simulink model "CRH2forBenchmark_Copy"  (R2014a)
settings: Solver=ode3  StartTime=0.0  StopTime=1  FixedStep=1e-5  RelTol=1e-3
PostLoadFcn:
  | , if any(exist('dsrtsu_mdlpostloadfcn', 'file') == [2, 3, 6]), try dsrtsu_mdlpostloadfcn('Execute', bdroot); catch fprintf('Error in PostLoadFcn (dsrtsu_mdlpostloadfcn) for model "%s":\n %s\n', bdroot, lasterr); end, end,
values from neighbouring files (symbols this model uses):
  Cd = 0.016    [CRH2forBenchmark.mat]
  Lm = 0.032848    [CRH2forBenchmark.mat]
  Ln = 0.002    [CRH2forBenchmark.mat]
  Lr = 0.034142    [CRH2forBenchmark.mat]
  Ls = 0.0342654    [CRH2forBenchmark.mat]
  np = 2    [CRH2forBenchmark.mat]
  Rd = 6000    [CRH2forBenchmark.mat]
  Rn = 0.2    [CRH2forBenchmark.mat]
  Rr = 0.146    [CRH2forBenchmark.mat]
  Rs = 0.144    [CRH2forBenchmark.mat]
  ts = 1e-05    [CRH2forBenchmark.mat]
undefined symbols (not defined in the file): J, KIM, KIT, KPM, KPT, phir, Ts, Vge
libraries: simulink x20
(part 3 of 5)

== system CRH2forBenchmark_Copy/Benchmark/SFI2/Subsystem ==
  Normal : Inport
  Outside Signal : Inport  Port=2
  Band-Limited White Noise : simulink/Sources/Band-Limited White Noise  Cov=NoiseFault(1)  Ts=NoiseFault(2)  seed=NoiseFault(3)
  Pulse Generator : DiscretePulseGenerator  PulseType=Time based  Amplitude=PeriodicFault(1)  Period=PeriodicFault(2)  PulseWidth=PeriodicFault(3)
  SFI1 : Subsystem  mask{sfcnParam1=AddMux, sfcnParam2=Comp_ConV, sfcnParam3=DriftFault, sfcnParam4=FaultCont, sfcnParam5=FaultInjectionTime, sfcnParam6=FaultType, sfcnParam7=NoiseSelec, sfcnParam8=ShockGain, sfcnParam9=Variance}
      mask prompts: sfcnParam1 "AddMux:"; sfcnParam2 "Comp_ConV:"; sfcnParam3 "DriftFault:"; sfcnParam4 "FaultCont:"; sfcnParam5 "FaultInjectionTime:"; sfcnParam6 "FaultType:"; sfcnParam7 "NoiseSelec:"; sfcnParam8 "ShockGain:"; sfcnParam9 "Variance:"
      mask help: Simulink:masks:GenSFuncDesc_MD
      mask Help: eval('feval(''rtwprivate'',''rtwhelpview'',''rtw_sfcn_block'')');
  Out : Outport
  tag scope: BandLimitedWhiteNoiseSFI2=global, PulseGeneratorSFI2=global
  wires:
  Band-Limited White Noise/1 -> [BandLimitedWhiteNoiseSFI2]
  Pulse Generator/1 -> [PulseGeneratorSFI2]
  Normal/1 -> SFI1/1(Nomal)
  Outside Signal/1 -> SFI1/2(Outside Signal)
  SFI1/1(Out) -> Out/1

== system CRH2forBenchmark_Copy/Benchmark/TFI1/TFI1Sub ==
  Nomal : Inport
  Outside Signal : Inport  Port=2
  Add : Sum
  Band-Limited White Noise : simulink/Sources/Band-Limited White Noise  Cov=NoiseFault(1)  Ts=NoiseFault(2)  seed=NoiseFault(3)
  Logic Operation : Subsystem
  Noise0 : Constant  Value=0
  NoiseAdd : Sum  Inputs=++|
  NoiseSelec : Constant  Value=NoiseSelec
  Product : Product
  Switch : Switch  Criteria=u2 ~= 0
  TFI : Subsystem
  Out : Outport
  wires:
  Outside Signal/1 -> TFI/1(Outside Signal)
  Switch/1 -> NoiseAdd/1
  Band-Limited White Noise/1 -> Switch/1
  [Fault] -> Logic Operation/5(Fault), Add/2, Product/2
  NoiseAdd/1 -> Out/1
  Logic Operation/1(Out) -> NoiseAdd/2
  Nomal/1 -> Add/1, Product/1, Logic Operation/4(Normal)
  Add/1 -> Logic Operation/2(Add)
  Noise0/1 -> Switch/3
  TFI/1(Fault Singal) -> [Fault]
  Product/1 -> Logic Operation/3(Mux)
  TFI/2(Selector) -> [Selector]
  [Selector] -> Logic Operation/1(Selector)
  NoiseSelec/1 -> Switch/2

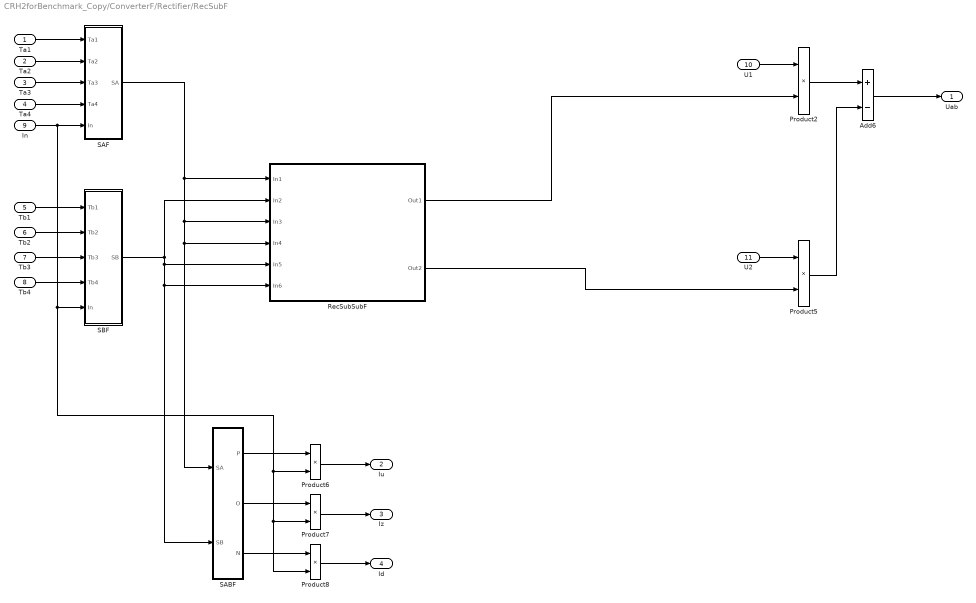
== system CRH2forBenchmark_Copy/ConverterF/Rectifier/RecSubF ==
  Ta1 : Inport
  Ta2 : Inport  Port=2
  Ta3 : Inport  Port=3
  Ta4 : Inport  Port=4
  Tb1 : Inport  Port=5
  Tb2 : Inport  Port=6
  Tb3 : Inport  Port=7
  Tb4 : Inport  Port=8
  In : Inport  Port=9
  U1 : Inport  Port=10
  U2 : Inport  Port=11
  Add6 : Sum  Inputs=+-  SampleTime=ts
  Product{2,5..8} (5 alike) : Product  SampleTime=ts
  RecSubSubF : Subsystem
      mask help: Simulink:masks:GenSFuncDesc_MD
      mask Help: eval('feval(''rtwprivate'',''rtwhelpview'',''rtw_sfcn_block'')');
  SABF : Subsystem
      mask help: Simulink:masks:GenSFuncDesc_MD
      mask Help: eval('feval(''rtwprivate'',''rtwhelpview'',''rtw_sfcn_block'')');
  SAF : Subsystem
      mask help: Simulink:masks:GenSFuncDesc_MD
      mask Help: eval('feval(''rtwprivate'',''rtwhelpview'',''rtw_sfcn_block'')');
  SBF : Subsystem
      mask help: Simulink:masks:GenSFuncDesc_MD
      mask Help: eval('feval(''rtwprivate'',''rtwhelpview'',''rtw_sfcn_block'')');
  Uab : Outport
  Iu : Outport  Port=2
  Iz : Outport  Port=3
  Id : Outport  Port=4
  wires:
  In/1 -> SAF/5(In), SBF/5(In), Product7/2, Product8/2, Product6/2
  Tb3/1 -> SBF/3(Tb3)
  U2/1 -> Product5/1
  Product2/1 -> Add6/1
  SAF/1(SA) -> RecSubSubF/1(In1), RecSubSubF/3(In3), RecSubSubF/4(In4), SABF/1(SA)
  U1/1 -> Product2/1
  Ta3/1 -> SAF/3(Ta3)
  Product5/1 -> Add6/2
  Tb1/1 -> SBF/1(Tb1)
  Add6/1 -> Uab/1
  Ta2/1 -> SAF/2(Ta2)
  Tb2/1 -> SBF/2(Tb2)
  SBF/1(SB) -> RecSubSubF/2(In2), RecSubSubF/5(In5), RecSubSubF/6(In6), SABF/2(SB)
  Tb4/1 -> SBF/4(Tb4)
  Ta1/1 -> SAF/1(Ta1)
  Ta4/1 -> SAF/4(Ta4)
  SABF/3(N) -> Product8/1
  SABF/2(O) -> Product7/1
  SABF/1(P) -> Product6/1
  Product6/1 -> Iu/1
  Product7/1 -> Iz/1
  Product8/1 -> Id/1
  RecSubSubF/1(Out1) -> Product2/2
  RecSubSubF/2(Out2) -> Product5/2

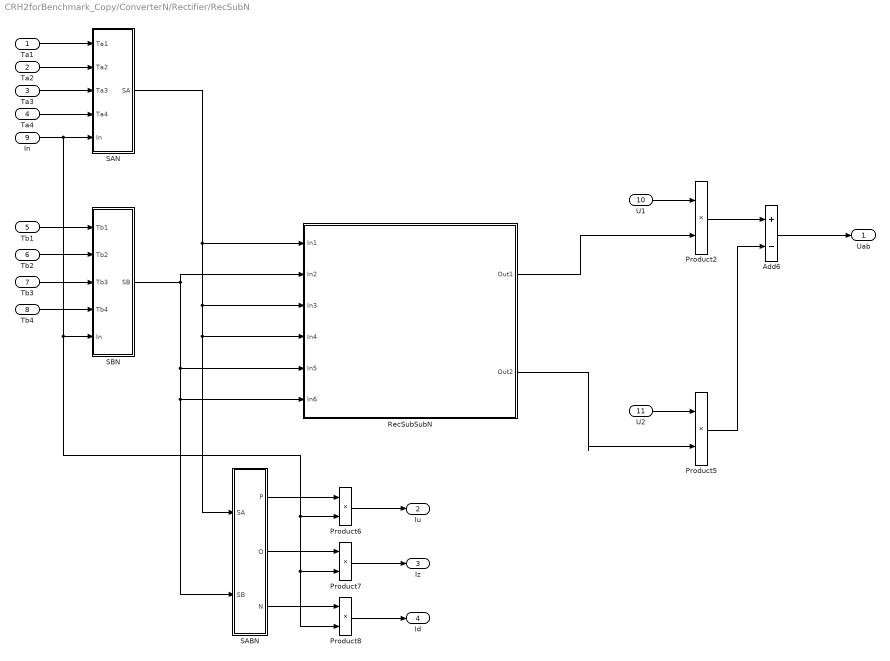
== system CRH2forBenchmark_Copy/ConverterN/Rectifier/RecSubN ==
  Ta1 : Inport
  Ta2 : Inport  Port=2
  Ta3 : Inport  Port=3
  Ta4 : Inport  Port=4
  Tb1 : Inport  Port=5
  Tb2 : Inport  Port=6
  Tb3 : Inport  Port=7
  Tb4 : Inport  Port=8
  In : Inport  Port=9
  U1 : Inport  Port=10
  U2 : Inport  Port=11
  Add6 : Sum  Inputs=+-  SampleTime=ts
  Product{2,5..8} (5 alike) : Product  SampleTime=ts
  RecSubSubN : Subsystem
      mask help: Simulink:masks:GenSFuncDesc_MD
      mask Help: eval('feval(''rtwprivate'',''rtwhelpview'',''rtw_sfcn_block'')');
  SABN : Subsystem
      mask help: Simulink:masks:GenSFuncDesc_MD
      mask Help: eval('feval(''rtwprivate'',''rtwhelpview'',''rtw_sfcn_block'')');
  SAN : Subsystem
      mask help: Simulink:masks:GenSFuncDesc_MD
      mask Help: eval('feval(''rtwprivate'',''rtwhelpview'',''rtw_sfcn_block'')');
  SBN : Subsystem
      mask help: Simulink:masks:GenSFuncDesc_MD
      mask Help: eval('feval(''rtwprivate'',''rtwhelpview'',''rtw_sfcn_block'')');
  Uab : Outport
  Iu : Outport  Port=2
  Iz : Outport  Port=3
  Id : Outport  Port=4
  wires:
  Product8/1 -> Id/1
  Product7/1 -> Iz/1
  Product6/1 -> Iu/1
  SABN/1(P) -> Product6/1
  SABN/2(O) -> Product7/1
  SABN/3(N) -> Product8/1
  Ta4/1 -> SAN/4(Ta4)
  Ta1/1 -> SAN/1(Ta1)
  Tb4/1 -> SBN/4(Tb4)
  SBN/1(SB) -> RecSubSubN/2(In2), RecSubSubN/5(In5), RecSubSubN/6(In6), SABN/2(SB)
  Tb2/1 -> SBN/2(Tb2)
  Ta2/1 -> SAN/2(Ta2)
  Add6/1 -> Uab/1
  Tb1/1 -> SBN/1(Tb1)
  Product5/1 -> Add6/2
  Ta3/1 -> SAN/3(Ta3)
  U1/1 -> Product2/1
  SAN/1(SA) -> RecSubSubN/1(In1), RecSubSubN/3(In3), RecSubSubN/4(In4), SABN/1(SA)
  Product2/1 -> Add6/1
  U2/1 -> Product5/1
  Tb3/1 -> SBN/3(Tb3)
  In/1 -> SAN/5(In), SBN/5(In), Product6/2, Product8/2, Product7/2
  RecSubSubN/1(Out1) -> Product2/2
  RecSubSubN/2(Out2) -> Product5/2

== system CRH2forBenchmark_Copy/InverterF/InverterTuF/__InputSSForSFun__ ==
  Tu1 : Inport
  Tu2 : Inport  Port=2
  Tu3 : Inport  Port=3
  Tu4 : Inport  Port=4
  Ia : Inport  Port=5
  U1 : Inport  Port=6
  U2 : Inport  Port=7
  __UniqueOutportName__1__ : Outport
  __UniqueOutportName__2__ : Outport  Port=2
  __UniqueOutportName__3__ : Outport  Port=3
  __UniqueOutportName__4__ : Outport  Port=4
  __UniqueOutportName__5__ : Outport  Port=5
  __UniqueOutportName__6__ : Outport  Port=6
  __UniqueOutportName__7__ : Outport  Port=7
  wires:
  Tu1/1 -> __UniqueOutportName__1__/1
  Tu2/1 -> __UniqueOutportName__2__/1
  Tu3/1 -> __UniqueOutportName__3__/1
  Tu4/1 -> __UniqueOutportName__4__/1
  Ia/1 -> __UniqueOutportName__5__/1
  U1/1 -> __UniqueOutportName__6__/1
  U2/1 -> __UniqueOutportName__7__/1

== system CRH2forBenchmark_Copy/InverterF/InverterTuF/__OutputSSForSFun__ ==
  __UniqueInportName__1__ : Inport
  __UniqueInportName__2__ : Inport  Port=2
  __UniqueInportName__3__ : Inport  Port=3
  __UniqueInportName__4__ : Inport  Port=4
  Iu : Outport
  Iz : Outport  Port=2
  Id : Outport  Port=3
  Vu : Outport  Port=4
  wires:
  __UniqueInportName__1__/1 -> Iu/1
  __UniqueInportName__2__/1 -> Iz/1
  __UniqueInportName__3__/1 -> Id/1
  __UniqueInportName__4__/1 -> Vu/1

== system CRH2forBenchmark_Copy/InverterF/InverterTvF/__InputSSForSFun__ ==
  Tv1 : Inport
  Tv2 : Inport  Port=2
  Tv3 : Inport  Port=3
  Tv4 : Inport  Port=4
  Ib : Inport  Port=5
  U1 : Inport  Port=6
  U2 : Inport  Port=7
  __UniqueOutportName__1__ : Outport
  __UniqueOutportName__2__ : Outport  Port=2
  __UniqueOutportName__3__ : Outport  Port=3
  __UniqueOutportName__4__ : Outport  Port=4
  __UniqueOutportName__5__ : Outport  Port=5
  __UniqueOutportName__6__ : Outport  Port=6
  __UniqueOutportName__7__ : Outport  Port=7
  wires:
  Tv1/1 -> __UniqueOutportName__1__/1
  Tv2/1 -> __UniqueOutportName__2__/1
  Tv3/1 -> __UniqueOutportName__3__/1
  Tv4/1 -> __UniqueOutportName__4__/1
  Ib/1 -> __UniqueOutportName__5__/1
  U1/1 -> __UniqueOutportName__6__/1
  U2/1 -> __UniqueOutportName__7__/1

== system CRH2forBenchmark_Copy/InverterF/InverterTvF/__OutputSSForSFun__ ==
  __UniqueInportName__1__ : Inport
  __UniqueInportName__2__ : Inport  Port=2
  __UniqueInportName__3__ : Inport  Port=3
  __UniqueInportName__4__ : Inport  Port=4
  Iu : Outport
  Iz : Outport  Port=2
  Id : Outport  Port=3
  Vv : Outport  Port=4
  wires:
  __UniqueInportName__1__/1 -> Iu/1
  __UniqueInportName__2__/1 -> Iz/1
  __UniqueInportName__3__/1 -> Id/1
  __UniqueInportName__4__/1 -> Vv/1

== system CRH2forBenchmark_Copy/InverterF/InverterTwF/__InputSSForSFun__ ==
  Tw1 : Inport
  Tw2 : Inport  Port=2
  Tw3 : Inport  Port=3
  Tw4 : Inport  Port=4
  Ic : Inport  Port=5
  U1 : Inport  Port=6
  U2 : Inport  Port=7
  __UniqueOutportName__1__ : Outport
  __UniqueOutportName__2__ : Outport  Port=2
  __UniqueOutportName__3__ : Outport  Port=3
  __UniqueOutportName__4__ : Outport  Port=4
  __UniqueOutportName__5__ : Outport  Port=5
  __UniqueOutportName__6__ : Outport  Port=6
  __UniqueOutportName__7__ : Outport  Port=7
  wires:
  Tw1/1 -> __UniqueOutportName__1__/1
  Tw2/1 -> __UniqueOutportName__2__/1
  Tw3/1 -> __UniqueOutportName__3__/1
  Tw4/1 -> __UniqueOutportName__4__/1
  Ic/1 -> __UniqueOutportName__5__/1
  U1/1 -> __UniqueOutportName__6__/1
  U2/1 -> __UniqueOutportName__7__/1

== system CRH2forBenchmark_Copy/InverterF/InverterTwF/__OutputSSForSFun__ ==
  __UniqueInportName__1__ : Inport
  __UniqueInportName__2__ : Inport  Port=2
  __UniqueInportName__3__ : Inport  Port=3
  __UniqueInportName__4__ : Inport  Port=4
  Iu : Outport
  Iz : Outport  Port=2
  Id : Outport  Port=3
  Vw : Outport  Port=4
  wires:
  __UniqueInportName__1__/1 -> Iu/1
  __UniqueInportName__2__/1 -> Iz/1
  __UniqueInportName__3__/1 -> Id/1
  __UniqueInportName__4__/1 -> Vw/1

== system CRH2forBenchmark_Copy/InverterN/InverterTuN/__InputSSForSFun__ ==
  Tu1 : Inport
  Tu2 : Inport  Port=2
  Tu3 : Inport  Port=3
  Tu4 : Inport  Port=4
  Ia : Inport  Port=5
  U1 : Inport  Port=6
  U2 : Inport  Port=7
  __UniqueOutportName__1__ : Outport
  __UniqueOutportName__2__ : Outport  Port=2
  __UniqueOutportName__3__ : Outport  Port=3
  __UniqueOutportName__4__ : Outport  Port=4
  __UniqueOutportName__5__ : Outport  Port=5
  __UniqueOutportName__6__ : Outport  Port=6
  __UniqueOutportName__7__ : Outport  Port=7
  wires:
  Tu1/1 -> __UniqueOutportName__1__/1
  Tu2/1 -> __UniqueOutportName__2__/1
  Tu3/1 -> __UniqueOutportName__3__/1
  Tu4/1 -> __UniqueOutportName__4__/1
  Ia/1 -> __UniqueOutportName__5__/1
  U1/1 -> __UniqueOutportName__6__/1
  U2/1 -> __UniqueOutportName__7__/1

== system CRH2forBenchmark_Copy/InverterN/InverterTuN/__OutputSSForSFun__ ==
  __UniqueInportName__1__ : Inport
  __UniqueInportName__2__ : Inport  Port=2
  __UniqueInportName__3__ : Inport  Port=3
  __UniqueInportName__4__ : Inport  Port=4
  Iu : Outport
  Iz : Outport  Port=2
  Id : Outport  Port=3
  Vu : Outport  Port=4
  wires:
  __UniqueInportName__1__/1 -> Iu/1
  __UniqueInportName__2__/1 -> Iz/1
  __UniqueInportName__3__/1 -> Id/1
  __UniqueInportName__4__/1 -> Vu/1

== system CRH2forBenchmark_Copy/InverterN/InverterTvN/__InputSSForSFun__ ==
  Tv1 : Inport
  Tv2 : Inport  Port=2
  Tv3 : Inport  Port=3
  Tv4 : Inport  Port=4
  Ib : Inport  Port=5
  U1 : Inport  Port=6
  U2 : Inport  Port=7
  __UniqueOutportName__1__ : Outport
  __UniqueOutportName__2__ : Outport  Port=2
  __UniqueOutportName__3__ : Outport  Port=3
  __UniqueOutportName__4__ : Outport  Port=4
  __UniqueOutportName__5__ : Outport  Port=5
  __UniqueOutportName__6__ : Outport  Port=6
  __UniqueOutportName__7__ : Outport  Port=7
  wires:
  Tv1/1 -> __UniqueOutportName__1__/1
  Tv2/1 -> __UniqueOutportName__2__/1
  Tv3/1 -> __UniqueOutportName__3__/1
  Tv4/1 -> __UniqueOutportName__4__/1
  Ib/1 -> __UniqueOutportName__5__/1
  U1/1 -> __UniqueOutportName__6__/1
  U2/1 -> __UniqueOutportName__7__/1

== system CRH2forBenchmark_Copy/InverterN/InverterTvN/__OutputSSForSFun__ ==
  __UniqueInportName__1__ : Inport
  __UniqueInportName__2__ : Inport  Port=2
  __UniqueInportName__3__ : Inport  Port=3
  __UniqueInportName__4__ : Inport  Port=4
  Iu : Outport
  Iz : Outport  Port=2
  Id : Outport  Port=3
  Vv : Outport  Port=4
  wires:
  __UniqueInportName__1__/1 -> Iu/1
  __UniqueInportName__2__/1 -> Iz/1
  __UniqueInportName__3__/1 -> Id/1
  __UniqueInportName__4__/1 -> Vv/1

== system CRH2forBenchmark_Copy/InverterN/InverterTwN/__InputSSForSFun__ ==
  Tw1 : Inport
  Tw2 : Inport  Port=2
  Tw3 : Inport  Port=3
  Tw4 : Inport  Port=4
  Ic : Inport  Port=5
  U1 : Inport  Port=6
  U2 : Inport  Port=7
  __UniqueOutportName__1__ : Outport
  __UniqueOutportName__2__ : Outport  Port=2
  __UniqueOutportName__3__ : Outport  Port=3
  __UniqueOutportName__4__ : Outport  Port=4
  __UniqueOutportName__5__ : Outport  Port=5
  __UniqueOutportName__6__ : Outport  Port=6
  __UniqueOutportName__7__ : Outport  Port=7
  wires:
  Tw1/1 -> __UniqueOutportName__1__/1
  Tw2/1 -> __UniqueOutportName__2__/1
  Tw3/1 -> __UniqueOutportName__3__/1
  Tw4/1 -> __UniqueOutportName__4__/1
  Ic/1 -> __UniqueOutportName__5__/1
  U1/1 -> __UniqueOutportName__6__/1
  U2/1 -> __UniqueOutportName__7__/1

== system CRH2forBenchmark_Copy/InverterN/InverterTwN/__OutputSSForSFun__ ==
  __UniqueInportName__1__ : Inport
  __UniqueInportName__2__ : Inport  Port=2
  __UniqueInportName__3__ : Inport  Port=3
  __UniqueInportName__4__ : Inport  Port=4
  Iu : Outport
  Iz : Outport  Port=2
  Id : Outport  Port=3
  Vw : Outport  Port=4
  wires:
  __UniqueInportName__1__/1 -> Iu/1
  __UniqueInportName__2__/1 -> Iz/1
  __UniqueInportName__3__/1 -> Id/1
  __UniqueInportName__4__/1 -> Vw/1

== system CRH2forBenchmark_Copy/Machine model/Normal ModelF/MeasurementF ==
  isα : Inport
  isβ : Inport  Port=2
  irα : Inport  Port=3
  irβ : Inport  Port=4
  TL : Inport  Port=5
  MeasurementF_sfcn : S-Function  FunctionName=MeasurementF_sf  Parameters=sfcnParam1, sfcnParam2, sfcnParam3  SFunctionModules=""  EnableBusSupport=off  mask{rtw_sf_name=MeasurementF_sf, showVar=off, sfcnParam1=sfcnParam1, sfcnParam2=sfcnParam2, sfcnParam3=sfcnParam3}
      mask prompts: rtw_sf_name "Simulink:masks:GenSFuncName_MP"; showVar "Simulink:masks:GenSFuncShowModuleList_MP"; sfcnParam1 "J:"; sfcnParam2 "Lm:"; sfcnParam3 "np:"
      mask help: Simulink:masks:GenSFuncDesc_MD
      mask init: same as CRH2forBenchmark_Copy/DCU1/DCU1_sfcn
      settings: CopyFcn=|
      | if ~strcmp(get_param(gcb,'Linkstatus'),'none') && ...
      | ~strcmp(get_param(gcb,'Linkstatus'),'implicit')
      |   set_param(gcb,'LinkStatus','none');
      | end
      mask Help: eval('feval(''rtwprivate'',''rtwhelpview'',''rtw_sfcn_block'')');
      mask Display:
      | port_label('input',1,'isα');
      | port_label('input',2,'isβ');
      | port_label('input',3,'irα');
      | port_label('input',4,'irβ');
      | port_label('input',5,'TL');
      | port_label('output',1,'Te');
      | port_label('output',2,'ω');
      | port_label('output',3,'Isabc');
  __InputSSForSFun__ : Subsystem
  __OutputSSForSFun__ : Subsystem
  Te : Outport
  ω : Outport  Port=2
  Isabc : Outport  Port=3
  wires:
  isα/1 -> __InputSSForSFun__/1(isα)
  isβ/1 -> __InputSSForSFun__/2(isβ)
  irα/1 -> __InputSSForSFun__/3(irα)
  irβ/1 -> __InputSSForSFun__/4(irβ)
  TL/1 -> __InputSSForSFun__/5(TL)
  __InputSSForSFun__/1(__UniqueOutportName__1__) -> MeasurementF_sfcn/1
  __InputSSForSFun__/2(__UniqueOutportName__2__) -> MeasurementF_sfcn/2
  __InputSSForSFun__/3(__UniqueOutportName__3__) -> MeasurementF_sfcn/3
  __InputSSForSFun__/4(__UniqueOutportName__4__) -> MeasurementF_sfcn/4
  __InputSSForSFun__/5(__UniqueOutportName__5__) -> MeasurementF_sfcn/5
  MeasurementF_sfcn/1 -> __OutputSSForSFun__/1(__UniqueInportName__1__)
  MeasurementF_sfcn/2 -> __OutputSSForSFun__/2(__UniqueInportName__2__)
  MeasurementF_sfcn/3 -> __OutputSSForSFun__/3(__UniqueInportName__3__)
  __OutputSSForSFun__/1(Te) -> Te/1
  __OutputSSForSFun__/2(ω) -> ω/1
  __OutputSSForSFun__/3(Isabc) -> Isabc/1

== system CRH2forBenchmark_Copy/Machine model/Normal ModelF/MotorSubsystem1F ==
  ψrβ : Inport
  Usβ : Inport  Port=2
  MotorSubsystem1FSub : Subsystem
  isβ : Outport
  ψsβ : Outport  Port=2
  wires:
  ψrβ/1 -> MotorSubsystem1FSub/1(ψrβ)
  Usβ/1 -> MotorSubsystem1FSub/2(Usβ)
  MotorSubsystem1FSub/1(isβ) -> isβ/1
  MotorSubsystem1FSub/2(ψsβ) -> ψsβ/1

== system CRH2forBenchmark_Copy/Machine model/Normal ModelF/MotorSubsystem2F ==
  ψsα : Inport
  ψrβ : Inport  Port=2
  ω : Inport  Port=3
  MotorSubsystem2FSub : Subsystem
  irα : Outport
  ψrα : Outport  Port=2
  wires:
  ψsα/1 -> MotorSubsystem2FSub/1(ψsα)
  ψrβ/1 -> MotorSubsystem2FSub/2(ψrβ)
  ω/1 -> MotorSubsystem2FSub/3(ω)
  MotorSubsystem2FSub/1(irα) -> irα/1
  MotorSubsystem2FSub/2(ψrα) -> ψrα/1

== system CRH2forBenchmark_Copy/Machine model/Normal ModelF/MotorSubsystem3F ==
  ψsβ : Inport
  ψrα : Inport  Port=2
  ω : Inport  Port=3
  MotorSubsystem3FSub : Subsystem
  irβ : Outport
  ψrβ : Outport  Port=2
  wires:
  ψsβ/1 -> MotorSubsystem3FSub/1(ψsβ)
  ψrα/1 -> MotorSubsystem3FSub/2(ψrα)
  ω/1 -> MotorSubsystem3FSub/3(ω)
  MotorSubsystem3FSub/1(irβ) -> irβ/1
  MotorSubsystem3FSub/2(ψrβ) -> ψrβ/1

== system CRH2forBenchmark_Copy/Machine model/Normal ModelF/MotorSubsystemF ==
  ψrα : Inport
  Usα : Inport  Port=2
  MotorSubsystemFSub : Subsystem
  isα : Outport
  ψsα : Outport  Port=2
  wires:
  ψrα/1 -> MotorSubsystemFSub/1(ψrα)
  Usα/1 -> MotorSubsystemFSub/2(Usα)
  MotorSubsystemFSub/1(isα) -> isα/1
  MotorSubsystemFSub/2(ψsα) -> ψsα/1

== system CRH2forBenchmark_Copy/Machine model/Normal ModelF/r2sF ==
  Ua : Inport
  Ub : Inport  Port=2
  Uc : Inport  Port=3
  __InputSSForSFun__ : Subsystem
  __OutputSSForSFun__ : Subsystem
  r2sF_sfcn : S-Function  FunctionName=r2sF_sf  SFunctionModules=""  EnableBusSupport=off  mask{rtw_sf_name=r2sF_sf, showVar=off}
      mask prompts: rtw_sf_name "Simulink:masks:GenSFuncName_MP"; showVar "Simulink:masks:GenSFuncShowModuleList_MP"
      mask help: Simulink:masks:GenSFuncDesc_MD
      mask init: same as CRH2forBenchmark_Copy/DCU1/DCU1_sfcn
      settings: CopyFcn=|
      | if ~strcmp(get_param(gcb,'Linkstatus'),'none') && ...
      | ~strcmp(get_param(gcb,'Linkstatus'),'implicit')
      |   set_param(gcb,'LinkStatus','none');
      | end
      mask Help: eval('feval(''rtwprivate'',''rtwhelpview'',''rtw_sfcn_block'')');
      mask Display:
      | port_label('input',1,'Ua');
      | port_label('input',2,'Ub');
      | port_label('input',3,'Uc');
      | port_label('output',1,'Usα');
      | port_label('output',2,'Usβ');
  Usα : Outport
  Usβ : Outport  Port=2
  wires:
  Ua/1 -> __InputSSForSFun__/1(Ua)
  Ub/1 -> __InputSSForSFun__/2(Ub)
  Uc/1 -> __InputSSForSFun__/3(Uc)
  __InputSSForSFun__/1(__UniqueOutportName__1__) -> r2sF_sfcn/1
  __InputSSForSFun__/2(__UniqueOutportName__2__) -> r2sF_sfcn/2
  __InputSSForSFun__/3(__UniqueOutportName__3__) -> r2sF_sfcn/3
  r2sF_sfcn/1 -> __OutputSSForSFun__/1(__UniqueInportName__1__)
  r2sF_sfcn/2 -> __OutputSSForSFun__/2(__UniqueInportName__2__)
  __OutputSSForSFun__/1(Usα) -> Usα/1
  __OutputSSForSFun__/2(Usβ) -> Usβ/1

== system CRH2forBenchmark_Copy/Machine model1/Normal ModelN/MeasurementN ==
  isα : Inport
  isβ : Inport  Port=2
  irα : Inport  Port=3
  irβ : Inport  Port=4
  TL : Inport  Port=5
  MeasurementN_sfcn : S-Function  FunctionName=MeasurementN_sf  Parameters=sfcnParam1, sfcnParam2, sfcnParam3  SFunctionModules=""  EnableBusSupport=off  mask{rtw_sf_name=MeasurementN_sf, showVar=off, sfcnParam1=sfcnParam1, sfcnParam2=sfcnParam2, sfcnParam3=sfcnParam3}
      mask prompts: rtw_sf_name "Simulink:masks:GenSFuncName_MP"; showVar "Simulink:masks:GenSFuncShowModuleList_MP"; sfcnParam1 "J:"; sfcnParam2 "Lm:"; sfcnParam3 "np:"
      mask help: Simulink:masks:GenSFuncDesc_MD
      mask init: same as CRH2forBenchmark_Copy/DCU1/DCU1_sfcn
      settings: CopyFcn=|
      | if ~strcmp(get_param(gcb,'Linkstatus'),'none') && ...
      | ~strcmp(get_param(gcb,'Linkstatus'),'implicit')
      |   set_param(gcb,'LinkStatus','none');
      | end
      mask Help: eval('feval(''rtwprivate'',''rtwhelpview'',''rtw_sfcn_block'')');
      mask Display:
      | port_label('input',1,'isα');
      | port_label('input',2,'isβ');
      | port_label('input',3,'irα');
      | port_label('input',4,'irβ');
      | port_label('input',5,'TL');
      | port_label('output',1,'Te');
      | port_label('output',2,'ω');
      | port_label('output',3,'Isabc');
  __InputSSForSFun__ : Subsystem
  __OutputSSForSFun__ : Subsystem
  Te : Outport
  ω : Outport  Port=2
  Isabc : Outport  Port=3
  wires:
  isα/1 -> __InputSSForSFun__/1(isα)
  isβ/1 -> __InputSSForSFun__/2(isβ)
  irα/1 -> __InputSSForSFun__/3(irα)
  irβ/1 -> __InputSSForSFun__/4(irβ)
  TL/1 -> __InputSSForSFun__/5(TL)
  __InputSSForSFun__/1(__UniqueOutportName__1__) -> MeasurementN_sfcn/1
  __InputSSForSFun__/2(__UniqueOutportName__2__) -> MeasurementN_sfcn/2
  __InputSSForSFun__/3(__UniqueOutportName__3__) -> MeasurementN_sfcn/3
  __InputSSForSFun__/4(__UniqueOutportName__4__) -> MeasurementN_sfcn/4
  __InputSSForSFun__/5(__UniqueOutportName__5__) -> MeasurementN_sfcn/5
  MeasurementN_sfcn/1 -> __OutputSSForSFun__/1(__UniqueInportName__1__)
  MeasurementN_sfcn/2 -> __OutputSSForSFun__/2(__UniqueInportName__2__)
  MeasurementN_sfcn/3 -> __OutputSSForSFun__/3(__UniqueInportName__3__)
  __OutputSSForSFun__/1(Te) -> Te/1
  __OutputSSForSFun__/2(ω) -> ω/1
  __OutputSSForSFun__/3(Isabc) -> Isabc/1

== system CRH2forBenchmark_Copy/Machine model1/Normal ModelN/MotorSubsystem1N ==
  ψrβ : Inport
  Usβ : Inport  Port=2
  MotorSubsystem1NSub : Subsystem
  isβ : Outport
  ψsβ : Outport  Port=2
  wires:
  ψrβ/1 -> MotorSubsystem1NSub/1(ψrβ)
  Usβ/1 -> MotorSubsystem1NSub/2(Usβ)
  MotorSubsystem1NSub/1(isβ) -> isβ/1
  MotorSubsystem1NSub/2(ψsβ) -> ψsβ/1

== system CRH2forBenchmark_Copy/Machine model1/Normal ModelN/MotorSubsystem2N ==
  ψsα : Inport
  ψrβ : Inport  Port=2
  ω : Inport  Port=3
  MotorSubsystem2NSub : Subsystem
  irα : Outport
  ψrα : Outport  Port=2
  wires:
  ψsα/1 -> MotorSubsystem2NSub/1(ψsα)
  ψrβ/1 -> MotorSubsystem2NSub/2(ψrβ)
  ω/1 -> MotorSubsystem2NSub/3(ω)
  MotorSubsystem2NSub/1(irα) -> irα/1
  MotorSubsystem2NSub/2(ψrα) -> ψrα/1

== system CRH2forBenchmark_Copy/Machine model1/Normal ModelN/MotorSubsystem3N ==
  ψsβ : Inport
  ψrα : Inport  Port=2
  ω : Inport  Port=3
  MotorSubsystem3NSub : Subsystem
  irβ : Outport
  ψrβ : Outport  Port=2
  wires:
  ψsβ/1 -> MotorSubsystem3NSub/1(ψsβ)
  ψrα/1 -> MotorSubsystem3NSub/2(ψrα)
  ω/1 -> MotorSubsystem3NSub/3(ω)
  MotorSubsystem3NSub/1(irβ) -> irβ/1
  MotorSubsystem3NSub/2(ψrβ) -> ψrβ/1

== system CRH2forBenchmark_Copy/Machine model1/Normal ModelN/MotorSubsystemN ==
  ψrα : Inport
  Usα : Inport  Port=2
  MotorSubsystemNSub : Subsystem
  isα : Outport
  ψsα : Outport  Port=2
  wires:
  ψrα/1 -> MotorSubsystemNSub/1(ψrα)
  Usα/1 -> MotorSubsystemNSub/2(Usα)
  MotorSubsystemNSub/1(isα) -> isα/1
  MotorSubsystemNSub/2(ψsα) -> ψsα/1

== system CRH2forBenchmark_Copy/Machine model1/Normal ModelN/r2sN ==
  Ua : Inport
  Ub : Inport  Port=2
  Uc : Inport  Port=3
  __InputSSForSFun__ : Subsystem
  __OutputSSForSFun__ : Subsystem
  r2sN_sfcn : S-Function  FunctionName=r2sN_sf  SFunctionModules=""  EnableBusSupport=off  mask{rtw_sf_name=r2sN_sf, showVar=off}
      mask prompts: rtw_sf_name "Simulink:masks:GenSFuncName_MP"; showVar "Simulink:masks:GenSFuncShowModuleList_MP"
      mask help: Simulink:masks:GenSFuncDesc_MD
      mask init: same as CRH2forBenchmark_Copy/DCU1/DCU1_sfcn
      settings: CopyFcn=|
      | if ~strcmp(get_param(gcb,'Linkstatus'),'none') && ...
      | ~strcmp(get_param(gcb,'Linkstatus'),'implicit')
      |   set_param(gcb,'LinkStatus','none');
      | end
      mask Help: eval('feval(''rtwprivate'',''rtwhelpview'',''rtw_sfcn_block'')');
      mask Display:
      | port_label('input',1,'Ua');
      | port_label('input',2,'Ub');
      | port_label('input',3,'Uc');
      | port_label('output',1,'Usα');
      | port_label('output',2,'Usβ');
  Usα : Outport
  Usβ : Outport  Port=2
  wires:
  Ua/1 -> __InputSSForSFun__/1(Ua)
  Ub/1 -> __InputSSForSFun__/2(Ub)
  Uc/1 -> __InputSSForSFun__/3(Uc)
  __InputSSForSFun__/1(__UniqueOutportName__1__) -> r2sN_sfcn/1
  __InputSSForSFun__/2(__UniqueOutportName__2__) -> r2sN_sfcn/2
  __InputSSForSFun__/3(__UniqueOutportName__3__) -> r2sN_sfcn/3
  r2sN_sfcn/1 -> __OutputSSForSFun__/1(__UniqueInportName__1__)
  r2sN_sfcn/2 -> __OutputSSForSFun__/2(__UniqueInportName__2__)
  __OutputSSForSFun__/1(Usα) -> Usα/1
  __OutputSSForSFun__/2(Usβ) -> Usβ/1

== system CRH2forBenchmark_Copy/Benchmark/CFI1/Subsystem2/Subsystem ==
  Clock : Clock
  Constant : Constant  Value=0
  Fault-States : Subsystem
  Gain : Gain  Gain=-1
  Multiport Switch2 : MultiPortSwitch  Inputs=4  DiagnosticForDefault=None
  N个频段的时间定位 : Subsystem
  Pulse Generator1 : DiscretePulseGenerator  PulseType=Time based  Period=ContantofPowerDevice(1,2)  PulseWidth=ContantofPowerDevice(1,3)  PhaseDelay=ContantofPowerDevice(1,4)
  Pulse Generator2 : DiscretePulseGenerator  PulseType=Time based  Period=ContantofPowerDevice(2,2)  PulseWidth=ContantofPowerDevice(2,3)  PhaseDelay=ContantofPowerDevice(2,4)
  Pulse Generator3 : DiscretePulseGenerator  PulseType=Time based  Period=ContantofPowerDevice(3,2)  PulseWidth=ContantofPowerDevice(3,3)  PhaseDelay=ContantofPowerDevice(3,4)
  Switch : Switch  Criteria=u2 > Threshold
  Periodic Signals : Outport
  wires:
  N个频段的时间定位/1(N) -> Multiport Switch2/1, Fault-States/1(In1)
  Fault-States/1(Out1) -> Switch/2
  Multiport Switch2/1 -> Gain/1, Switch/1
  Gain/1 -> Switch/3
  Switch/1 -> Periodic Signals/1
  Pulse Generator1/1 -> Multiport Switch2/3
  Pulse Generator2/1 -> Multiport Switch2/4
  Pulse Generator3/1 -> Multiport Switch2/5
  Constant/1 -> Multiport Switch2/2
  Clock/1 -> N个频段的时间定位/1(Timer)

== system CRH2forBenchmark_Copy/Benchmark/CFI1/Subsystem2/Subsystem1 ==
  Nomal : Inport
  Outside Signal1 : Inport  Port=2
  Subsystem1_sfcn : S-Function  FunctionName=Subsystem1_sf  Parameters=sfcnParam1, sfcnParam2, sfcnParam3, sfcnParam4, sfcnParam5, sfcnParam6  SFunctionModules=""  EnableBusSupport=off  mask{rtw_sf_name=Subsystem1_sf, showVar=off, sfcnParam1=sfcnParam1, sfcnParam2=sfcnParam2, sfcnParam3=sfcnParam3, sfcnParam4=sfcnParam4, sfcnParam5=sfcnParam5, sfcnParam6=sfcnParam6}
      mask prompts: rtw_sf_name "Simulink:masks:GenSFuncName_MP"; showVar "Simulink:masks:GenSFuncShowModuleList_MP"; sfcnParam1 "AddMux:"; sfcnParam2 "ContantofPassiveDevice:"; sfcnParam3 "FaultInjectionTime:"; sfcnParam4 "FaultType:"; sfcnParam5 "NoiseSelec:"; sfcnParam6 "PerformanceDegradationValue:"
      mask help: Simulink:masks:GenSFuncDesc_MD
      mask init: same as CRH2forBenchmark_Copy/DCU1/DCU1_sfcn
      settings: CopyFcn=|
      | if ~strcmp(get_param(gcb,'Linkstatus'),'none') && ...
      | ~strcmp(get_param(gcb,'Linkstatus'),'implicit')
      |   set_param(gcb,'LinkStatus','none');
      | end
      mask Help: eval('feval(''rtwprivate'',''rtwhelpview'',''rtw_sfcn_block'')');
      mask Display:
      | port_label('input',1,'Nomal');
      | port_label('input',2,'Outside Signal1');
      | port_label('input',3,'Inport1');
      | port_label('input',4,'Inport2');
      | port_label('output',1,'Out');
  __InputSSForSFun__ : Subsystem
  __OutputSSForSFun__ : Subsystem
  Out : Outport
  wires:
  __OutputSSForSFun__/1(Out) -> Out/1
  Subsystem1_sfcn/1 -> __OutputSSForSFun__/1(__UniqueInportName__1__)
  __InputSSForSFun__/4(__UniqueOutportName__4__) -> Subsystem1_sfcn/4
  __InputSSForSFun__/3(__UniqueOutportName__3__) -> Subsystem1_sfcn/3
  __InputSSForSFun__/2(__UniqueOutportName__2__) -> Subsystem1_sfcn/2
  __InputSSForSFun__/1(__UniqueOutportName__1__) -> Subsystem1_sfcn/1
  Outside Signal1/1 -> __InputSSForSFun__/2(Outside Signal1)
  Nomal/1 -> __InputSSForSFun__/1(Nomal)

== system CRH2forBenchmark_Copy/Benchmark/CFI2/Subsystem2/Subsystem ==
  Clock : Clock
  Constant : Constant  Value=0
  Fault-States : Subsystem
  Gain : Gain  Gain=-1
  Multiport Switch2 : MultiPortSwitch  Inputs=4  DiagnosticForDefault=None
  N个频段的时间定位 : Subsystem
  Pulse Generator1 : DiscretePulseGenerator  PulseType=Time based  Period=ContantofPowerDevice(1,2)  PulseWidth=ContantofPowerDevice(1,3)  PhaseDelay=ContantofPowerDevice(1,4)
  Pulse Generator2 : DiscretePulseGenerator  PulseType=Time based  Period=ContantofPowerDevice(2,2)  PulseWidth=ContantofPowerDevice(2,3)  PhaseDelay=ContantofPowerDevice(2,4)
  Pulse Generator3 : DiscretePulseGenerator  PulseType=Time based  Period=ContantofPowerDevice(3,2)  PulseWidth=ContantofPowerDevice(3,3)  PhaseDelay=ContantofPowerDevice(3,4)
  Switch : Switch  Criteria=u2 > Threshold
  Periodic Signals : Outport
  wires:
  N个频段的时间定位/1(N) -> Multiport Switch2/1, Fault-States/1(In1)
  Fault-States/1(Out1) -> Switch/2
  Multiport Switch2/1 -> Gain/1, Switch/1
  Gain/1 -> Switch/3
  Switch/1 -> Periodic Signals/1
  Pulse Generator1/1 -> Multiport Switch2/3
  Pulse Generator2/1 -> Multiport Switch2/4
  Pulse Generator3/1 -> Multiport Switch2/5
  Constant/1 -> Multiport Switch2/2
  Clock/1 -> N个频段的时间定位/1(Timer)

== system CRH2forBenchmark_Copy/Benchmark/CFI2/Subsystem2/Subsystem1 ==
  Nomal : Inport
  Outside Signal1 : Inport  Port=2
  Subsystem1_sfcn : S-Function  FunctionName=Subsystem1_sf  Parameters=sfcnParam1, sfcnParam2, sfcnParam3, sfcnParam4, sfcnParam5, sfcnParam6  SFunctionModules=""  EnableBusSupport=off  mask{rtw_sf_name=Subsystem1_sf, showVar=off, sfcnParam1=sfcnParam1, sfcnParam2=sfcnParam2, sfcnParam3=sfcnParam3, sfcnParam4=sfcnParam4, sfcnParam5=sfcnParam5, sfcnParam6=sfcnParam6}
      mask prompts: rtw_sf_name "Simulink:masks:GenSFuncName_MP"; showVar "Simulink:masks:GenSFuncShowModuleList_MP"; sfcnParam1 "AddMux:"; sfcnParam2 "ContantofPassiveDevice:"; sfcnParam3 "FaultInjectionTime:"; sfcnParam4 "FaultType:"; sfcnParam5 "NoiseSelec:"; sfcnParam6 "PerformanceDegradationValue:"
      mask help: Simulink:masks:GenSFuncDesc_MD
      mask init: same as CRH2forBenchmark_Copy/DCU1/DCU1_sfcn
      settings: CopyFcn=|
      | if ~strcmp(get_param(gcb,'Linkstatus'),'none') && ...
      | ~strcmp(get_param(gcb,'Linkstatus'),'implicit')
      |   set_param(gcb,'LinkStatus','none');
      | end
      mask Help: eval('feval(''rtwprivate'',''rtwhelpview'',''rtw_sfcn_block'')');
      mask Display:
      | port_label('input',1,'Nomal');
      | port_label('input',2,'Outside Signal1');
      | port_label('input',3,'Inport1');
      | port_label('input',4,'Inport2');
      | port_label('output',1,'Out');
  __InputSSForSFun__ : Subsystem
  __OutputSSForSFun__ : Subsystem
  Out : Outport
  wires:
  __OutputSSForSFun__/1(Out) -> Out/1
  Subsystem1_sfcn/1 -> __OutputSSForSFun__/1(__UniqueInportName__1__)
  __InputSSForSFun__/4(__UniqueOutportName__4__) -> Subsystem1_sfcn/4
  __InputSSForSFun__/3(__UniqueOutportName__3__) -> Subsystem1_sfcn/3
  __InputSSForSFun__/2(__UniqueOutportName__2__) -> Subsystem1_sfcn/2
  __InputSSForSFun__/1(__UniqueOutportName__1__) -> Subsystem1_sfcn/1
  Outside Signal1/1 -> __InputSSForSFun__/2(Outside Signal1)
  Nomal/1 -> __InputSSForSFun__/1(Nomal)

== system CRH2forBenchmark_Copy/Benchmark/MFI1/MFI1/MFI  ==
  Normal : Inport
  OutsideSignal : Inport  Port=2
  Band-Limited White Noise : simulink/Sources/Band-Limited White Noise  Cov=NoiseFault(1)  Ts=NoiseFault(2)  seed=NoiseFault(3)
  MFI1 : Subsystem  mask{sfcnParam1=AddMux, sfcnParam2=BearingFP, sfcnParam3=FS, sfcnParam4=FaultInjectionTime, sfcnParam5=FaultType, sfcnParam6=NoiseSelec, sfcnParam7=Severity1, sfcnParam8=Severity2, sfcnParam9=Severity3}
      mask prompts: sfcnParam1 "AddMux:"; sfcnParam2 "BearingFP:"; sfcnParam3 "FS:"; sfcnParam4 "FaultInjectionTime:"; sfcnParam5 "FaultType:"; sfcnParam6 "NoiseSelec:"; sfcnParam7 "Severity1:"; sfcnParam8 "Severity2:"; sfcnParam9 "Severity3:"
      mask help: Simulink:masks:GenSFuncDesc_MD
      mask Help: eval('feval(''rtwprivate'',''rtwhelpview'',''rtw_sfcn_block'')');
  Out : Outport
  tag scope: NoiseMFI1=global
  wires:
  Band-Limited White Noise/1 -> [NoiseMFI1]
  MFI1/1(Out) -> Out/1
  Normal/1 -> MFI1/1(Nomal)
  OutsideSignal/1 -> MFI1/2(Outside Signal1)

== system CRH2forBenchmark_Copy/Benchmark/MFI1/MFI2/MFI  ==
  Normal : Inport
  OutsideSignal : Inport  Port=2
  Band-Limited White Noise : simulink/Sources/Band-Limited White Noise  Cov=NoiseFault(1)  Ts=NoiseFault(2)  seed=NoiseFault(3)
  MFI1 : Subsystem  mask{sfcnParam1=AddMux, sfcnParam2=BearingFP, sfcnParam3=FS, sfcnParam4=FaultInjectionTime, sfcnParam5=FaultType, sfcnParam6=NoiseSelec, sfcnParam7=Severity1, sfcnParam8=Severity2, sfcnParam9=Severity3}
      mask prompts: sfcnParam1 "AddMux:"; sfcnParam2 "BearingFP:"; sfcnParam3 "FS:"; sfcnParam4 "FaultInjectionTime:"; sfcnParam5 "FaultType:"; sfcnParam6 "NoiseSelec:"; sfcnParam7 "Severity1:"; sfcnParam8 "Severity2:"; sfcnParam9 "Severity3:"
      mask help: Simulink:masks:GenSFuncDesc_MD
      mask Help: eval('feval(''rtwprivate'',''rtwhelpview'',''rtw_sfcn_block'')');
  Out : Outport
  tag scope: NoiseMFI2=global
  wires:
  OutsideSignal/1 -> MFI1/2(Outside Signal1)
  Normal/1 -> MFI1/1(Nomal)
  MFI1/1(Out) -> Out/1
  Band-Limited White Noise/1 -> [NoiseMFI2]

== system CRH2forBenchmark_Copy/Benchmark/MFI1/MFI3/MFI  ==
  Normal : Inport
  OutsideSignal : Inport  Port=2
  Band-Limited White Noise : simulink/Sources/Band-Limited White Noise  Cov=NoiseFault(1)  Ts=NoiseFault(2)  seed=NoiseFault(3)
  MFI1 : Subsystem  mask{sfcnParam1=AddMux, sfcnParam2=BearingFP, sfcnParam3=FS, sfcnParam4=FaultInjectionTime, sfcnParam5=FaultType, sfcnParam6=NoiseSelec, sfcnParam7=Severity1, sfcnParam8=Severity2, sfcnParam9=Severity3}
      mask prompts: sfcnParam1 "AddMux:"; sfcnParam2 "BearingFP:"; sfcnParam3 "FS:"; sfcnParam4 "FaultInjectionTime:"; sfcnParam5 "FaultType:"; sfcnParam6 "NoiseSelec:"; sfcnParam7 "Severity1:"; sfcnParam8 "Severity2:"; sfcnParam9 "Severity3:"
      mask help: Simulink:masks:GenSFuncDesc_MD
      mask Help: eval('feval(''rtwprivate'',''rtwhelpview'',''rtw_sfcn_block'')');
  Out : Outport
  tag scope: NoiseMFI3=global
  wires:
  Band-Limited White Noise/1 -> [NoiseMFI3]
  MFI1/1(Out) -> Out/1
  Normal/1 -> MFI1/1(Nomal)
  OutsideSignal/1 -> MFI1/2(Outside Signal1)

== system CRH2forBenchmark_Copy/Benchmark/MFI1/MFI4/MFI  ==
  Normal : Inport
  OutsideSignal : Inport  Port=2
  Band-Limited White Noise : simulink/Sources/Band-Limited White Noise  Cov=NoiseFault(1)  Ts=NoiseFault(2)  seed=NoiseFault(3)
  MFI1 : Subsystem  mask{sfcnParam1=AddMux, sfcnParam2=BearingFP, sfcnParam3=FS, sfcnParam4=FaultInjectionTime, sfcnParam5=FaultType, sfcnParam6=NoiseSelec, sfcnParam7=Severity1, sfcnParam8=Severity2, sfcnParam9=Severity3}
      mask prompts: sfcnParam1 "AddMux:"; sfcnParam2 "BearingFP:"; sfcnParam3 "FS:"; sfcnParam4 "FaultInjectionTime:"; sfcnParam5 "FaultType:"; sfcnParam6 "NoiseSelec:"; sfcnParam7 "Severity1:"; sfcnParam8 "Severity2:"; sfcnParam9 "Severity3:"
      mask help: Simulink:masks:GenSFuncDesc_MD
      mask Help: eval('feval(''rtwprivate'',''rtwhelpview'',''rtw_sfcn_block'')');
  Out : Outport
  tag scope: NoiseMFI4=global
  wires:
  Band-Limited White Noise/1 -> [NoiseMFI4]
  MFI1/1(Out) -> Out/1
  Normal/1 -> MFI1/1(Nomal)
  OutsideSignal/1 -> MFI1/2(Outside Signal1)

== system CRH2forBenchmark_Copy/Benchmark/MFI1/MFI5/MFI  ==
  Normal : Inport
  OutsideSignal : Inport  Port=2
  Band-Limited White Noise : simulink/Sources/Band-Limited White Noise  Cov=NoiseFault(1)  Ts=NoiseFault(2)  seed=NoiseFault(3)
  MFI1 : Subsystem  mask{sfcnParam1=AddMux, sfcnParam2=BearingFP, sfcnParam3=FS, sfcnParam4=FaultInjectionTime, sfcnParam5=FaultType, sfcnParam6=NoiseSelec, sfcnParam7=Severity1, sfcnParam8=Severity2, sfcnParam9=Severity3}
      mask prompts: sfcnParam1 "AddMux:"; sfcnParam2 "BearingFP:"; sfcnParam3 "FS:"; sfcnParam4 "FaultInjectionTime:"; sfcnParam5 "FaultType:"; sfcnParam6 "NoiseSelec:"; sfcnParam7 "Severity1:"; sfcnParam8 "Severity2:"; sfcnParam9 "Severity3:"
      mask help: Simulink:masks:GenSFuncDesc_MD
      mask Help: eval('feval(''rtwprivate'',''rtwhelpview'',''rtw_sfcn_block'')');
  Out : Outport
  tag scope: NoiseMFI5=global
  wires:
  OutsideSignal/1 -> MFI1/2(Outside Signal1)
  Normal/1 -> MFI1/1(Nomal)
  MFI1/1(Out) -> Out/1
  Band-Limited White Noise/1 -> [NoiseMFI5]

== system CRH2forBenchmark_Copy/Benchmark/MFI1/MFI6/MFI  ==
  Normal : Inport
  OutsideSignal : Inport  Port=2
  Band-Limited White Noise : simulink/Sources/Band-Limited White Noise  Cov=NoiseFault(1)  Ts=NoiseFault(2)  seed=NoiseFault(3)
  MFI1 : Subsystem  mask{sfcnParam1=AddMux, sfcnParam2=BearingFP, sfcnParam3=FS, sfcnParam4=FaultInjectionTime, sfcnParam5=FaultType, sfcnParam6=NoiseSelec, sfcnParam7=Severity1, sfcnParam8=Severity2, sfcnParam9=Severity3}
      mask prompts: sfcnParam1 "AddMux:"; sfcnParam2 "BearingFP:"; sfcnParam3 "FS:"; sfcnParam4 "FaultInjectionTime:"; sfcnParam5 "FaultType:"; sfcnParam6 "NoiseSelec:"; sfcnParam7 "Severity1:"; sfcnParam8 "Severity2:"; sfcnParam9 "Severity3:"
      mask help: Simulink:masks:GenSFuncDesc_MD
      mask Help: eval('feval(''rtwprivate'',''rtwhelpview'',''rtw_sfcn_block'')');
  Out : Outport
  tag scope: NoiseMFI6=global
  wires:
  OutsideSignal/1 -> MFI1/2(Outside Signal1)
  Normal/1 -> MFI1/1(Nomal)
  MFI1/1(Out) -> Out/1
  Band-Limited White Noise/1 -> [NoiseMFI6]

== system CRH2forBenchmark_Copy/Benchmark/SFI1/Subsystem/SFI1 ==
  Nomal : Inport
  Outside Signal : Inport  Port=2
  SFI_sfcn : S-Function  FunctionName=SFI0_sf  Parameters=sfcnParam1, sfcnParam2, sfcnParam3, sfcnParam4, sfcnParam5, sfcnParam6, sfcnParam7, sfcnParam8, sfcnParam9  SFunctionModules=""  EnableBusSupport=off  mask{rtw_sf_name=SFI0_sf, showVar=off, sfcnParam1=sfcnParam1, sfcnParam2=sfcnParam2, sfcnParam3=sfcnParam3, sfcnParam4=sfcnParam4, sfcnParam5=sfcnParam5, sfcnParam6=sfcnParam6, sfcnParam7=sfcnParam7, sfcnParam8=sfcnParam8, sfcnParam9=sfcnParam9}
      mask prompts: rtw_sf_name "Simulink:masks:GenSFuncName_MP"; showVar "Simulink:masks:GenSFuncShowModuleList_MP"; sfcnParam1 "AddMux:"; sfcnParam2 "Comp_ConV:"; sfcnParam3 "DriftFault:"; sfcnParam4 "FaultCont:"; sfcnParam5 "FaultInjectionTime:"; sfcnParam6 "FaultType:"; sfcnParam7 "NoiseSelec:"; sfcnParam8 "ShockGain:"; sfcnParam9 "Variance:"
      mask help: Simulink:masks:GenSFuncDesc_MD
      mask init: same as CRH2forBenchmark_Copy/DCU1/DCU1_sfcn
      settings: CopyFcn=|
      | if ~strcmp(get_param(gcb,'Linkstatus'),'none') && ...
      | ~strcmp(get_param(gcb,'Linkstatus'),'implicit')
      |   set_param(gcb,'LinkStatus','none');
      | end
      mask Help: eval('feval(''rtwprivate'',''rtwhelpview'',''rtw_sfcn_block'')');
      mask Display:
      | port_label('input',1,'Nomal');
      | port_label('input',2,'Outside Signal');
      | port_label('input',3,'Inport1');
      | port_label('input',4,'Inport2');
      | port_label('output',1,'Out');
  __InputSSForSFun__ : Subsystem
  __OutputSSForSFun__ : Subsystem
  Out : Outport
  wires:
  Nomal/1 -> __InputSSForSFun__/1(Nomal)
  Outside Signal/1 -> __InputSSForSFun__/2(Outside Signal)
  __InputSSForSFun__/1(__UniqueOutportName__1__) -> SFI_sfcn/1
  __InputSSForSFun__/2(__UniqueOutportName__2__) -> SFI_sfcn/2
  __InputSSForSFun__/3(__UniqueOutportName__3__) -> SFI_sfcn/3
  __InputSSForSFun__/4(__UniqueOutportName__4__) -> SFI_sfcn/4
  SFI_sfcn/1 -> __OutputSSForSFun__/1(__UniqueInportName__1__)
  __OutputSSForSFun__/1(Out) -> Out/1

== system CRH2forBenchmark_Copy/Benchmark/SFI2/Subsystem/SFI1 ==
  Nomal : Inport
  Outside Signal : Inport  Port=2
  SFI_sfcn : S-Function  FunctionName=SFI0_sf  Parameters=sfcnParam1, sfcnParam2, sfcnParam3, sfcnParam4, sfcnParam5, sfcnParam6, sfcnParam7, sfcnParam8, sfcnParam9  SFunctionModules=""  EnableBusSupport=off  mask{rtw_sf_name=SFI0_sf, showVar=off, sfcnParam1=sfcnParam1, sfcnParam2=sfcnParam2, sfcnParam3=sfcnParam3, sfcnParam4=sfcnParam4, sfcnParam5=sfcnParam5, sfcnParam6=sfcnParam6, sfcnParam7=sfcnParam7, sfcnParam8=sfcnParam8, sfcnParam9=sfcnParam9}
      mask prompts: rtw_sf_name "Simulink:masks:GenSFuncName_MP"; showVar "Simulink:masks:GenSFuncShowModuleList_MP"; sfcnParam1 "AddMux:"; sfcnParam2 "Comp_ConV:"; sfcnParam3 "DriftFault:"; sfcnParam4 "FaultCont:"; sfcnParam5 "FaultInjectionTime:"; sfcnParam6 "FaultType:"; sfcnParam7 "NoiseSelec:"; sfcnParam8 "ShockGain:"; sfcnParam9 "Variance:"
      mask help: Simulink:masks:GenSFuncDesc_MD
      mask init: same as CRH2forBenchmark_Copy/DCU1/DCU1_sfcn
      settings: CopyFcn=|
      | if ~strcmp(get_param(gcb,'Linkstatus'),'none') && ...
      | ~strcmp(get_param(gcb,'Linkstatus'),'implicit')
      |   set_param(gcb,'LinkStatus','none');
      | end
      mask Help: eval('feval(''rtwprivate'',''rtwhelpview'',''rtw_sfcn_block'')');
      mask Display:
      | port_label('input',1,'Nomal');
      | port_label('input',2,'Outside Signal');
      | port_label('input',3,'Inport1');
      | port_label('input',4,'Inport2');
      | port_label('output',1,'Out');
  __InputSSForSFun__ : Subsystem
  __OutputSSForSFun__ : Subsystem
  Out : Outport
  wires:
  Nomal/1 -> __InputSSForSFun__/1(Nomal)
  Outside Signal/1 -> __InputSSForSFun__/2(Outside Signal)
  __InputSSForSFun__/1(__UniqueOutportName__1__) -> SFI_sfcn/1
  __InputSSForSFun__/2(__UniqueOutportName__2__) -> SFI_sfcn/2
  __InputSSForSFun__/3(__UniqueOutportName__3__) -> SFI_sfcn/3
  __InputSSForSFun__/4(__UniqueOutportName__4__) -> SFI_sfcn/4
  SFI_sfcn/1 -> __OutputSSForSFun__/1(__UniqueInportName__1__)
  __OutputSSForSFun__/1(Out) -> Out/1

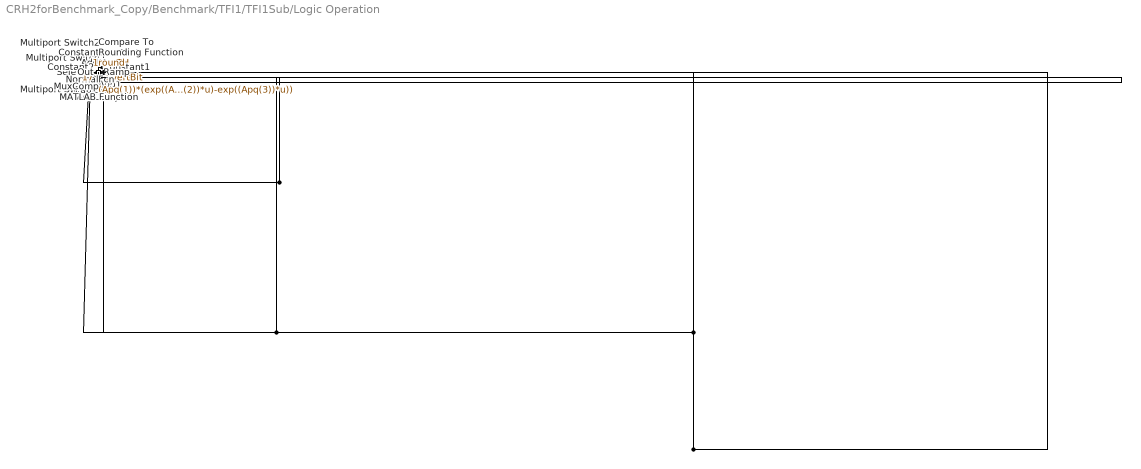
== system CRH2forBenchmark_Copy/Benchmark/TFI1/TFI1Sub/Logic Operation ==
  Selector : Inport
  Add : Inport  Port=2
  Mux : Inport  Port=3
  Normal : Inport  Port=4
  Fault : Inport  Port=5
  Add1 : Sum  Inputs=+-
  AddComp : Subsystem
  Compare To Constant : simulink/Logic and Bit Operations/Compare To Constant  relop=>=  const=TH  OutDataTypeStr=boolean
  Constant : Constant
  Constant1 : Constant  Value=InvertBit
  Constant2 : Constant  Value=17
  FaultSelec : Step  Time=FaultInjectionTime  Before=1  After=FaultType  SampleTime=0
  Fcn : Fcn  Expr=(Apq(1))*(exp((Apq(2))*u)-exp((Apq(3))*u))
  MATLAB Function : MATLAB Function  TreatAsAtomicUnit=on  SystemSampleTime=Register_Ts
  Multiport Switch : MultiPortSwitch  DataPortOrder=Zero-based contiguous  Inputs=2
  Multiport Switch1 : MultiPortSwitch  DataPortOrder=Specify indices  Inputs=2  DataPortIndices={[1,2,5],3,4}
  Multiport Switch2 : MultiPortSwitch  Inputs=8
  MuxComp : Subsystem
  Ramp : simulink/Sources/Ramp  slope=1  start=FaultInjectionTime  X0=0
  Rounding Function : Rounding  Operator=round  SampleTime=Register_Ts
  Out : Outport
  wires:
  Mux/1 -> MuxComp/1(Mux), Multiport Switch2/5
  Selector/1 -> Multiport Switch2/1
  Add/1 -> AddComp/1(Add), Multiport Switch2/2
  Multiport Switch1/1 -> Out/1
  FaultSelec/1 -> Multiport Switch1/1
  Multiport Switch2/1 -> Rounding Function/1, Multiport Switch/2, Multiport Switch1/2
  Constant/1 -> Multiport Switch/3
  Ramp/1 -> Fcn/1
  Fcn/1 -> Compare To Constant/1
  Compare To Constant/1 -> Multiport Switch/1
  Multiport Switch/1 -> Multiport Switch1/3
  Normal/1 -> Multiport Switch2/8
  AddComp/1(Out1) -> Multiport Switch2/3
  AddComp/2(Out2) -> Multiport Switch2/4
  MuxComp/1(Out1) -> Multiport Switch2/6
  MuxComp/2(Out2) -> Multiport Switch2/7
  Rounding Function/1 -> MATLAB Function/1(x)
  Constant1/1 -> Add1/2
  MATLAB Function/1(y) -> Multiport Switch1/4
  Add1/1 -> MATLAB Function/2(Num)
  Constant2/1 -> Add1/1
  Fault/1 -> Multiport Switch2/9

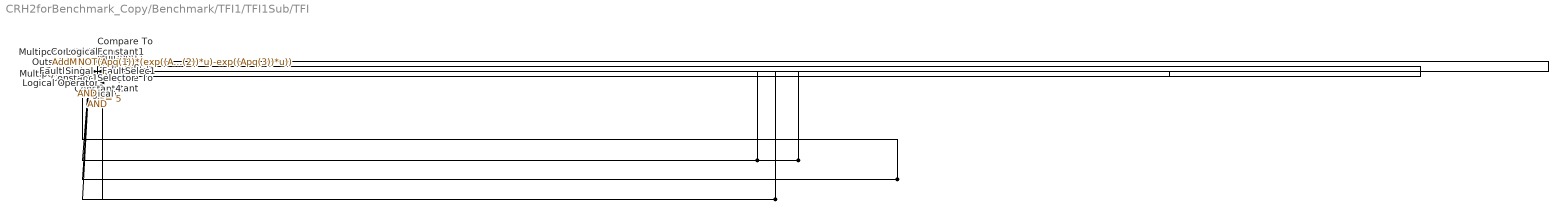
== system CRH2forBenchmark_Copy/Benchmark/TFI1/TFI1Sub/TFI ==
  Outside Signal : Inport
  " " : Constant  Value=7
  "  " : Constant
  "   " : Constant  Value=4
  "   1" : Constant  Value=8
  0 : Constant  Value=0
  Compare To Constant : simulink/Logic and Bit Operations/Compare To Constant  relop===  const=5  OutDataTypeStr=boolean
  Compare To Constant1 : simulink/Logic and Bit Operations/Compare To Constant  relop===  const=5  OutDataTypeStr=boolean
  Constant1 : Constant  Value=5
  Constant2 : Constant  Value=AddMux-1
  Constant3 : Constant  Value=2
  Constant4 : Constant  Value=6
  FaultSelec : Step  Time=FaultInjectionTime  Before=1  After=FaultType  SampleTime=0
  FaultSelec1 : Step  Time=FaultInjectionTime  Before=1  After=FaultType  SampleTime=0
  Fcn : Fcn  Expr=(Apq(1))*(exp((Apq(2))*u)-exp((Apq(3))*u))
  Logical : Logic  Operator=NOT  AllPortsSameDT=off  OutDataTypeStr=boolean
  "Logical " : Logic  AllPortsSameDT=off  OutDataTypeStr=boolean
  Logical Operator : Logic  AllPortsSameDT=off  OutDataTypeStr=boolean
  Multiport : MultiPortSwitch  DataPortOrder=Zero-based contiguous  Inputs=2
  Multiport Switch : MultiPortSwitch  DataPortOrder=Specify indices  Inputs=4  DataPortIndices={[1,3,4],2,5}
  Multiport Switch1 : MultiPortSwitch  DataPortOrder=Specify indices  Inputs=4  DataPortIndices={[1,3,4],2,5,6}
  "Multiport  " : MultiPortSwitch  DataPortOrder=Zero-based contiguous  Inputs=2
  Multiport1 : MultiPortSwitch  DataPortOrder=Zero-based contiguous  Inputs=2
  Ramp : simulink/Sources/Ramp  slope=1  start=FaultInjectionTime  X0=0
  Fault Singal : Outport
  Selector : Outport  Port=2
  wires:
  Ramp/1 -> Fcn/1
  Multiport Switch/1 -> Fault Singal/1
  FaultSelec/1 -> Multiport Switch/1
  Multiport Switch1/1 -> Selector/1
  0/1 -> Multiport Switch/2
  Fcn/1 -> Multiport Switch/3
  " "/1 -> Multiport Switch1/2
  "  "/1 -> Multiport Switch1/3
  FaultSelec1/1 -> Compare To Constant/1, Multiport/2
  Constant2/1 -> Compare To Constant1/1, Logical/1, Logical Operator/1
  Compare To Constant/1 -> "Logical "/2, Logical Operator/2
  Logical Operator/1 -> Multiport/1
  Multiport1/1 -> Multiport/3
  "Multiport  "/1 -> Multiport Switch1/1
  Constant3/1 -> "Multiport  "/3
  Multiport/1 -> "Multiport  "/2
  "Logical "/1 -> "Multiport  "/1
  Logical/1 -> "Logical "/1
  "   "/1 -> Multiport Switch1/4
  Outside Signal/1 -> Multiport Switch/4
  Compare To Constant1/1 -> Multiport1/1
  Constant4/1 -> Multiport1/3
  Constant1/1 -> Multiport1/2
  "   1"/1 -> Multiport Switch1/5

== system CRH2forBenchmark_Copy/ConverterF/Rectifier/RecSubF/RecSubSubF ==
  In1 : Inport
  In2 : Inport  Port=2
  In3 : Inport  Port=3
  In4 : Inport  Port=4
  In5 : Inport  Port=5
  In6 : Inport  Port=6
  RecSubSubF_sfcn : S-Function  FunctionName=RecSubSubF_sf  SFunctionModules=""  EnableBusSupport=off  mask{rtw_sf_name=RecSubSubF_sf, showVar=off}
      mask prompts: rtw_sf_name "Simulink:masks:GenSFuncName_MP"; showVar "Simulink:masks:GenSFuncShowModuleList_MP"
      mask help: Simulink:masks:GenSFuncDesc_MD
      mask init: same as CRH2forBenchmark_Copy/DCU1/DCU1_sfcn
      settings: CopyFcn=|
      | if ~strcmp(get_param(gcb,'Linkstatus'),'none') && ...
      | ~strcmp(get_param(gcb,'Linkstatus'),'implicit')
      |   set_param(gcb,'LinkStatus','none');
      | end
      mask Help: eval('feval(''rtwprivate'',''rtwhelpview'',''rtw_sfcn_block'')');
      mask Display:
      | port_label('input',1,'In1');
      | port_label('input',2,'In2');
      | port_label('input',3,'In3');
      | port_label('input',4,'In4');
      | port_label('input',5,'In5');
      | port_label('input',6,'In6');
      | port_label('output',1,'Out1');
      | port_label('output',2,'Out2');
  __InputSSForSFun__ : Subsystem
  __OutputSSForSFun__ : Subsystem
  Out1 : Outport
  Out2 : Outport  Port=2
  wires:
  In1/1 -> __InputSSForSFun__/1(In1)
  In2/1 -> __InputSSForSFun__/2(In2)
  In3/1 -> __InputSSForSFun__/3(In3)
  In4/1 -> __InputSSForSFun__/4(In4)
  In5/1 -> __InputSSForSFun__/5(In5)
  In6/1 -> __InputSSForSFun__/6(In6)
  __InputSSForSFun__/1(__UniqueOutportName__1__) -> RecSubSubF_sfcn/1
  __InputSSForSFun__/2(__UniqueOutportName__2__) -> RecSubSubF_sfcn/2
  __InputSSForSFun__/3(__UniqueOutportName__3__) -> RecSubSubF_sfcn/3
  __InputSSForSFun__/4(__UniqueOutportName__4__) -> RecSubSubF_sfcn/4
  __InputSSForSFun__/5(__UniqueOutportName__5__) -> RecSubSubF_sfcn/5
  __InputSSForSFun__/6(__UniqueOutportName__6__) -> RecSubSubF_sfcn/6
  RecSubSubF_sfcn/1 -> __OutputSSForSFun__/1(__UniqueInportName__1__)
  RecSubSubF_sfcn/2 -> __OutputSSForSFun__/2(__UniqueInportName__2__)
  __OutputSSForSFun__/1(Out1) -> Out1/1
  __OutputSSForSFun__/2(Out2) -> Out2/1
